simulink model "large_scale_autosar_swc_expfcns"  (R2021a)
settings: Solver=FixedStepDiscrete  StartTime=0.0  StopTime=20  FixedStep=1  MaxStep=.0001  RelTol=1e-3  EnableMultiTasking=on
undefined symbols (not defined in the file): DiscIntNeverNeededParam
(part 2 of 3)

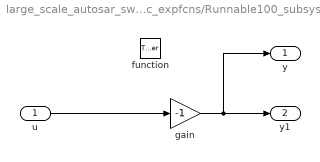
== system large_scale_autosar_swc_expfcns/Runnable100_subsystem ==
  u : Inport
  function : TriggerPort  TriggerType=function-call  VariantControl=Variant  SampleTimeType=periodic  SampleTime=-1
  gain : Gain  Gain=-1  ParamDataTypeStr=int8  OutDataTypeStr=int8
  y : Outport  InitialOutput=0  VectorParamsAs1DForOutWhenUnconnected=off
  y1 : Outport  Port=2  VectorParamsAs1DForOutWhenUnconnected=off
  wires:
  u/1 -> gain/1
  gain/1 -> y/1, y1/1

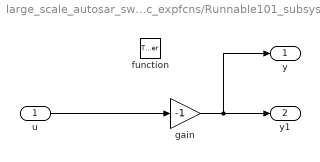
== system large_scale_autosar_swc_expfcns/Runnable101_subsystem ==
  u : Inport
  function : TriggerPort  TriggerType=function-call  VariantControl=Variant  SampleTimeType=periodic  SampleTime=-1
  gain : Gain  Gain=-1  ParamDataTypeStr=int8  OutDataTypeStr=int8
  y : Outport  InitialOutput=0  VectorParamsAs1DForOutWhenUnconnected=off
  y1 : Outport  Port=2  VectorParamsAs1DForOutWhenUnconnected=off
  wires:
  u/1 -> gain/1
  gain/1 -> y/1, y1/1

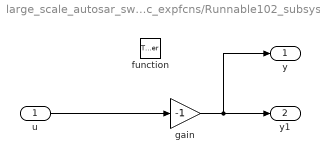
== system large_scale_autosar_swc_expfcns/Runnable102_subsystem ==
  u : Inport
  function : TriggerPort  TriggerType=function-call  VariantControl=Variant  SampleTimeType=periodic  SampleTime=-1
  gain : Gain  Gain=-1  ParamDataTypeStr=int8  OutDataTypeStr=int8
  y : Outport  InitialOutput=0  VectorParamsAs1DForOutWhenUnconnected=off
  y1 : Outport  Port=2  VectorParamsAs1DForOutWhenUnconnected=off
  wires:
  u/1 -> gain/1
  gain/1 -> y/1, y1/1

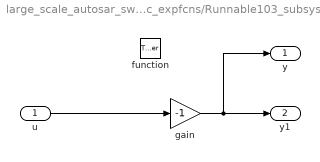
== system large_scale_autosar_swc_expfcns/Runnable103_subsystem ==
  u : Inport
  function : TriggerPort  TriggerType=function-call  VariantControl=Variant  SampleTimeType=periodic  SampleTime=-1
  gain : Gain  Gain=-1  ParamDataTypeStr=int8  OutDataTypeStr=int8
  y : Outport  InitialOutput=0  VectorParamsAs1DForOutWhenUnconnected=off
  y1 : Outport  Port=2  VectorParamsAs1DForOutWhenUnconnected=off
  wires:
  u/1 -> gain/1
  gain/1 -> y/1, y1/1

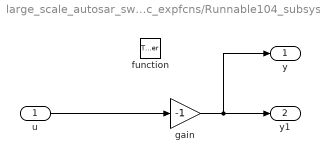
== system large_scale_autosar_swc_expfcns/Runnable104_subsystem ==
  u : Inport
  function : TriggerPort  TriggerType=function-call  VariantControl=Variant  SampleTimeType=periodic  SampleTime=-1
  gain : Gain  Gain=-1  ParamDataTypeStr=int8  OutDataTypeStr=int8
  y : Outport  InitialOutput=0  VectorParamsAs1DForOutWhenUnconnected=off
  y1 : Outport  Port=2  VectorParamsAs1DForOutWhenUnconnected=off
  wires:
  u/1 -> gain/1
  gain/1 -> y/1, y1/1

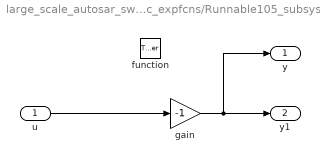
== system large_scale_autosar_swc_expfcns/Runnable105_subsystem ==
  u : Inport
  function : TriggerPort  TriggerType=function-call  VariantControl=Variant  SampleTimeType=periodic  SampleTime=-1
  gain : Gain  Gain=-1  ParamDataTypeStr=int8  OutDataTypeStr=int8
  y : Outport  InitialOutput=0  VectorParamsAs1DForOutWhenUnconnected=off
  y1 : Outport  Port=2  VectorParamsAs1DForOutWhenUnconnected=off
  wires:
  u/1 -> gain/1
  gain/1 -> y/1, y1/1

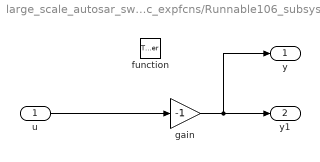
== system large_scale_autosar_swc_expfcns/Runnable106_subsystem ==
  u : Inport
  function : TriggerPort  TriggerType=function-call  VariantControl=Variant  SampleTimeType=periodic  SampleTime=-1
  gain : Gain  Gain=-1  ParamDataTypeStr=int8  OutDataTypeStr=int8
  y : Outport  InitialOutput=0  VectorParamsAs1DForOutWhenUnconnected=off
  y1 : Outport  Port=2  VectorParamsAs1DForOutWhenUnconnected=off
  wires:
  u/1 -> gain/1
  gain/1 -> y/1, y1/1

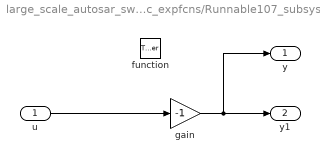
== system large_scale_autosar_swc_expfcns/Runnable107_subsystem ==
  u : Inport
  function : TriggerPort  TriggerType=function-call  VariantControl=Variant  SampleTimeType=periodic  SampleTime=-1
  gain : Gain  Gain=-1  ParamDataTypeStr=int8  OutDataTypeStr=int8
  y : Outport  InitialOutput=0  VectorParamsAs1DForOutWhenUnconnected=off
  y1 : Outport  Port=2  VectorParamsAs1DForOutWhenUnconnected=off
  wires:
  u/1 -> gain/1
  gain/1 -> y/1, y1/1

== system large_scale_autosar_swc_expfcns/Runnable108_subsystem ==
  u : Inport
  function : TriggerPort  TriggerType=function-call  VariantControl=Variant  SampleTimeType=periodic  SampleTime=-1
  gain : Gain  Gain=-1  ParamDataTypeStr=int8  OutDataTypeStr=int8
  y : Outport  InitialOutput=0  VectorParamsAs1DForOutWhenUnconnected=off
  y1 : Outport  Port=2  VectorParamsAs1DForOutWhenUnconnected=off
  wires:
  u/1 -> gain/1
  gain/1 -> y/1, y1/1

== system large_scale_autosar_swc_expfcns/Runnable10_subsystem ==
  u : Inport
  function : TriggerPort  TriggerType=function-call  VariantControl=Variant  SampleTimeType=periodic  SampleTime=-1
  gain : Gain  Gain=-1  ParamDataTypeStr=int8  OutDataTypeStr=int8
  y : Outport  InitialOutput=0  VectorParamsAs1DForOutWhenUnconnected=off
  y1 : Outport  Port=2  VectorParamsAs1DForOutWhenUnconnected=off
  wires:
  u/1 -> gain/1
  gain/1 -> y/1, y1/1

== system large_scale_autosar_swc_expfcns/Runnable11_subsystem ==
  u : Inport
  function : TriggerPort  TriggerType=function-call  VariantControl=Variant  SampleTimeType=periodic  SampleTime=-1
  gain : Gain  Gain=-1  ParamDataTypeStr=int8  OutDataTypeStr=int8
  y : Outport  InitialOutput=0  VectorParamsAs1DForOutWhenUnconnected=off
  y1 : Outport  Port=2  VectorParamsAs1DForOutWhenUnconnected=off
  wires:
  u/1 -> gain/1
  gain/1 -> y/1, y1/1

== system large_scale_autosar_swc_expfcns/Runnable12_subsystem ==
  u : Inport
  function : TriggerPort  TriggerType=function-call  VariantControl=Variant  SampleTimeType=periodic  SampleTime=-1
  gain : Gain  Gain=-1  ParamDataTypeStr=int8  OutDataTypeStr=int8
  y : Outport  InitialOutput=0  VectorParamsAs1DForOutWhenUnconnected=off
  y1 : Outport  Port=2  VectorParamsAs1DForOutWhenUnconnected=off
  wires:
  u/1 -> gain/1
  gain/1 -> y/1, y1/1

== system large_scale_autosar_swc_expfcns/Runnable13_subsystem ==
  u : Inport
  function : TriggerPort  TriggerType=function-call  VariantControl=Variant  SampleTimeType=periodic  SampleTime=-1
  gain : Gain  Gain=-1  ParamDataTypeStr=int8  OutDataTypeStr=int8
  y : Outport  InitialOutput=0  VectorParamsAs1DForOutWhenUnconnected=off
  y1 : Outport  Port=2  VectorParamsAs1DForOutWhenUnconnected=off
  wires:
  u/1 -> gain/1
  gain/1 -> y/1, y1/1

== system large_scale_autosar_swc_expfcns/Runnable14_subsystem ==
  u : Inport
  function : TriggerPort  TriggerType=function-call  VariantControl=Variant  SampleTimeType=periodic  SampleTime=-1
  gain : Gain  Gain=-1  ParamDataTypeStr=int8  OutDataTypeStr=int8
  y : Outport  InitialOutput=0  VectorParamsAs1DForOutWhenUnconnected=off
  y1 : Outport  Port=2  VectorParamsAs1DForOutWhenUnconnected=off
  wires:
  u/1 -> gain/1
  gain/1 -> y/1, y1/1

== system large_scale_autosar_swc_expfcns/Runnable15_subsystem ==
  u : Inport
  function : TriggerPort  TriggerType=function-call  VariantControl=Variant  SampleTimeType=periodic  SampleTime=-1
  gain : Gain  Gain=-1  ParamDataTypeStr=int8  OutDataTypeStr=int8
  y : Outport  InitialOutput=0  VectorParamsAs1DForOutWhenUnconnected=off
  y1 : Outport  Port=2  VectorParamsAs1DForOutWhenUnconnected=off
  wires:
  u/1 -> gain/1
  gain/1 -> y/1, y1/1

== system large_scale_autosar_swc_expfcns/Runnable16_subsystem ==
  u : Inport
  function : TriggerPort  TriggerType=function-call  VariantControl=Variant  SampleTimeType=periodic  SampleTime=-1
  gain : Gain  Gain=-1  ParamDataTypeStr=int8  OutDataTypeStr=int8
  y : Outport  InitialOutput=0  VectorParamsAs1DForOutWhenUnconnected=off
  y1 : Outport  Port=2  VectorParamsAs1DForOutWhenUnconnected=off
  wires:
  u/1 -> gain/1
  gain/1 -> y/1, y1/1

== system large_scale_autosar_swc_expfcns/Runnable17_subsystem ==
  u : Inport
  function : TriggerPort  TriggerType=function-call  VariantControl=Variant  SampleTimeType=periodic  SampleTime=-1
  gain : Gain  Gain=-1  ParamDataTypeStr=int8  OutDataTypeStr=int8
  y : Outport  InitialOutput=0  VectorParamsAs1DForOutWhenUnconnected=off
  y1 : Outport  Port=2  VectorParamsAs1DForOutWhenUnconnected=off
  wires:
  u/1 -> gain/1
  gain/1 -> y/1, y1/1

== system large_scale_autosar_swc_expfcns/Runnable18_subsystem ==
  u : Inport
  function : TriggerPort  TriggerType=function-call  VariantControl=Variant  SampleTimeType=periodic  SampleTime=-1
  gain : Gain  Gain=-1  ParamDataTypeStr=int8  OutDataTypeStr=int8
  y : Outport  InitialOutput=0  VectorParamsAs1DForOutWhenUnconnected=off
  y1 : Outport  Port=2  VectorParamsAs1DForOutWhenUnconnected=off
  wires:
  u/1 -> gain/1
  gain/1 -> y/1, y1/1

== system large_scale_autosar_swc_expfcns/Runnable19_subsystem ==
  u : Inport
  function : TriggerPort  TriggerType=function-call  VariantControl=Variant  SampleTimeType=periodic  SampleTime=-1
  gain : Gain  Gain=-1  ParamDataTypeStr=int8  OutDataTypeStr=int8
  y : Outport  InitialOutput=0  VectorParamsAs1DForOutWhenUnconnected=off
  y1 : Outport  Port=2  VectorParamsAs1DForOutWhenUnconnected=off
  wires:
  u/1 -> gain/1
  gain/1 -> y/1, y1/1

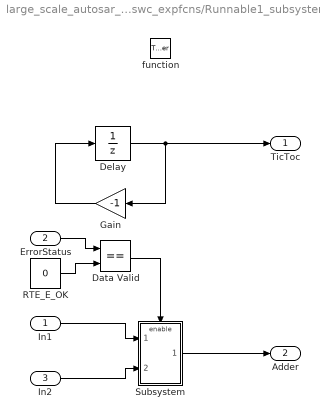
== system large_scale_autosar_swc_expfcns/Runnable1_subsystem ==
  In1 : Inport
  ErrorStatus : Inport  Port=2
  In2 : Inport  Port=3
  function : TriggerPort  TriggerType=function-call  VariantControl=Variant  SampleTimeType=periodic  SampleTime=-1
  Data Valid : RelationalOperator  Operator===  OutDataTypeStr=boolean  RndMeth=Nearest
  Delay : UnitDelay  InitialCondition=1  SampleTime=-1  HasFrameUpgradeWarning=on
  Gain : Gain  Gain=-1  OutDataTypeStr=fixdt(1,8,0)
  RTE_E_OK : Constant  Value=0
  Subsystem : Subsystem
  TicToc : Outport  InitialOutput=0  VectorParamsAs1DForOutWhenUnconnected=off
  Adder : Outport  Port=2  InitialOutput=0  VectorParamsAs1DForOutWhenUnconnected=off
  wires:
  RTE_E_OK/1 -> Data Valid/2
  ErrorStatus/1 -> Data Valid/1
  Data Valid/1 -> Subsystem/Enable
  In2/1 -> Subsystem/2(In2)
  In1/1 -> Subsystem/1(In1)
  Delay/1 -> Gain/1, TicToc/1
  Gain/1 -> Delay/1
  Subsystem/1(Adder) -> Adder/1

== system large_scale_autosar_swc_expfcns/Runnable20_subsystem ==
  u : Inport
  function : TriggerPort  TriggerType=function-call  VariantControl=Variant  SampleTimeType=periodic  SampleTime=-1
  gain : Gain  Gain=-1  ParamDataTypeStr=int8  OutDataTypeStr=int8
  y : Outport  InitialOutput=0  VectorParamsAs1DForOutWhenUnconnected=off
  y1 : Outport  Port=2  VectorParamsAs1DForOutWhenUnconnected=off
  wires:
  u/1 -> gain/1
  gain/1 -> y/1, y1/1

== system large_scale_autosar_swc_expfcns/Runnable21_subsystem ==
  u : Inport
  function : TriggerPort  TriggerType=function-call  VariantControl=Variant  SampleTimeType=periodic  SampleTime=-1
  gain : Gain  Gain=-1  ParamDataTypeStr=int8  OutDataTypeStr=int8
  y : Outport  InitialOutput=0  VectorParamsAs1DForOutWhenUnconnected=off
  y1 : Outport  Port=2  VectorParamsAs1DForOutWhenUnconnected=off
  wires:
  u/1 -> gain/1
  gain/1 -> y/1, y1/1

== system large_scale_autosar_swc_expfcns/Runnable22_subsystem ==
  u : Inport
  function : TriggerPort  TriggerType=function-call  VariantControl=Variant  SampleTimeType=periodic  SampleTime=-1
  gain : Gain  Gain=-1  ParamDataTypeStr=int8  OutDataTypeStr=int8
  y : Outport  InitialOutput=0  VectorParamsAs1DForOutWhenUnconnected=off
  y1 : Outport  Port=2  VectorParamsAs1DForOutWhenUnconnected=off
  wires:
  u/1 -> gain/1
  gain/1 -> y/1, y1/1

== system large_scale_autosar_swc_expfcns/Runnable23_subsystem ==
  u : Inport
  function : TriggerPort  TriggerType=function-call  VariantControl=Variant  SampleTimeType=periodic  SampleTime=-1
  gain : Gain  Gain=-1  ParamDataTypeStr=int8  OutDataTypeStr=int8
  y : Outport  InitialOutput=0  VectorParamsAs1DForOutWhenUnconnected=off
  y1 : Outport  Port=2  VectorParamsAs1DForOutWhenUnconnected=off
  wires:
  u/1 -> gain/1
  gain/1 -> y/1, y1/1

== system large_scale_autosar_swc_expfcns/Runnable24_subsystem ==
  u : Inport
  function : TriggerPort  TriggerType=function-call  VariantControl=Variant  SampleTimeType=periodic  SampleTime=-1
  gain : Gain  Gain=-1  ParamDataTypeStr=int8  OutDataTypeStr=int8
  y : Outport  InitialOutput=0  VectorParamsAs1DForOutWhenUnconnected=off
  y1 : Outport  Port=2  VectorParamsAs1DForOutWhenUnconnected=off
  wires:
  u/1 -> gain/1
  gain/1 -> y/1, y1/1

== system large_scale_autosar_swc_expfcns/Runnable25_subsystem ==
  u : Inport
  function : TriggerPort  TriggerType=function-call  VariantControl=Variant  SampleTimeType=periodic  SampleTime=-1
  gain : Gain  Gain=-1  ParamDataTypeStr=int8  OutDataTypeStr=int8
  y : Outport  InitialOutput=0  VectorParamsAs1DForOutWhenUnconnected=off
  y1 : Outport  Port=2  VectorParamsAs1DForOutWhenUnconnected=off
  wires:
  u/1 -> gain/1
  gain/1 -> y/1, y1/1

== system large_scale_autosar_swc_expfcns/Runnable26_subsystem ==
  u : Inport
  function : TriggerPort  TriggerType=function-call  VariantControl=Variant  SampleTimeType=periodic  SampleTime=-1
  gain : Gain  Gain=-1  ParamDataTypeStr=int8  OutDataTypeStr=int8
  y : Outport  InitialOutput=0  VectorParamsAs1DForOutWhenUnconnected=off
  y1 : Outport  Port=2  VectorParamsAs1DForOutWhenUnconnected=off
  wires:
  u/1 -> gain/1
  gain/1 -> y/1, y1/1

== system large_scale_autosar_swc_expfcns/Runnable27_subsystem ==
  u : Inport
  function : TriggerPort  TriggerType=function-call  VariantControl=Variant  SampleTimeType=periodic  SampleTime=-1
  gain : Gain  Gain=-1  ParamDataTypeStr=int8  OutDataTypeStr=int8
  y : Outport  InitialOutput=0  VectorParamsAs1DForOutWhenUnconnected=off
  y1 : Outport  Port=2  VectorParamsAs1DForOutWhenUnconnected=off
  wires:
  u/1 -> gain/1
  gain/1 -> y/1, y1/1

== system large_scale_autosar_swc_expfcns/Runnable28_subsystem ==
  u : Inport
  function : TriggerPort  TriggerType=function-call  VariantControl=Variant  SampleTimeType=periodic  SampleTime=-1
  gain : Gain  Gain=-1  ParamDataTypeStr=int8  OutDataTypeStr=int8
  y : Outport  InitialOutput=0  VectorParamsAs1DForOutWhenUnconnected=off
  y1 : Outport  Port=2  VectorParamsAs1DForOutWhenUnconnected=off
  wires:
  u/1 -> gain/1
  gain/1 -> y/1, y1/1

== system large_scale_autosar_swc_expfcns/Runnable29_subsystem ==
  u : Inport
  function : TriggerPort  TriggerType=function-call  VariantControl=Variant  SampleTimeType=periodic  SampleTime=-1
  gain : Gain  Gain=-1  ParamDataTypeStr=int8  OutDataTypeStr=int8
  y : Outport  InitialOutput=0  VectorParamsAs1DForOutWhenUnconnected=off
  y1 : Outport  Port=2  VectorParamsAs1DForOutWhenUnconnected=off
  wires:
  u/1 -> gain/1
  gain/1 -> y/1, y1/1

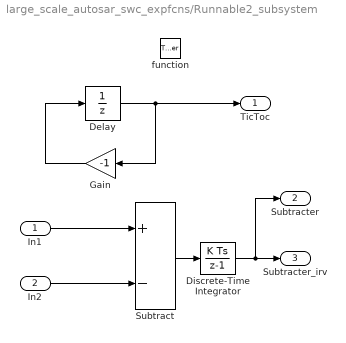
== system large_scale_autosar_swc_expfcns/Runnable2_subsystem ==
  In1 : Inport
  In2 : Inport  Port=2
  function : TriggerPort  TriggerType=function-call  VariantControl=Variant  SampleTimeType=periodic  SampleTime=-1
  Delay : UnitDelay  InitialCondition=1  SampleTime=-1  HasFrameUpgradeWarning=on
  Discrete-Time Integrator : DiscreteIntegrator  SampleTime=-1  ICPrevOutput=DiscIntNeverNeededParam  ICPrevScaledInput=DiscIntNeverNeededParam
  Gain : Gain  Gain=-1  OutDataTypeStr=fixdt(1,8,0)
  Subtract : Sum  Inputs=+-
  TicToc : Outport  InitialOutput=0  VectorParamsAs1DForOutWhenUnconnected=off
  Subtracter : Outport  Port=2  InitialOutput=0  VectorParamsAs1DForOutWhenUnconnected=off
  Subtracter_irv : Outport  Port=3  VectorParamsAs1DForOutWhenUnconnected=off
  wires:
  Discrete-Time Integrator/1 -> Subtracter/1, Subtracter_irv/1
  Subtract/1 -> Discrete-Time Integrator/1
  Gain/1 -> Delay/1
  Delay/1 -> TicToc/1, Gain/1
  In1/1 -> Subtract/1
  In2/1 -> Subtract/2

== system large_scale_autosar_swc_expfcns/Runnable30_subsystem ==
  u : Inport
  function : TriggerPort  TriggerType=function-call  VariantControl=Variant  SampleTimeType=periodic  SampleTime=-1
  gain : Gain  Gain=-1  ParamDataTypeStr=int8  OutDataTypeStr=int8
  y : Outport  InitialOutput=0  VectorParamsAs1DForOutWhenUnconnected=off
  y1 : Outport  Port=2  VectorParamsAs1DForOutWhenUnconnected=off
  wires:
  u/1 -> gain/1
  gain/1 -> y/1, y1/1

== system large_scale_autosar_swc_expfcns/Runnable31_subsystem ==
  u : Inport
  function : TriggerPort  TriggerType=function-call  VariantControl=Variant  SampleTimeType=periodic  SampleTime=-1
  gain : Gain  Gain=-1  ParamDataTypeStr=int8  OutDataTypeStr=int8
  y : Outport  InitialOutput=0  VectorParamsAs1DForOutWhenUnconnected=off
  y1 : Outport  Port=2  VectorParamsAs1DForOutWhenUnconnected=off
  wires:
  u/1 -> gain/1
  gain/1 -> y/1, y1/1

== system large_scale_autosar_swc_expfcns/Runnable32_subsystem ==
  u : Inport
  function : TriggerPort  TriggerType=function-call  VariantControl=Variant  SampleTimeType=periodic  SampleTime=-1
  gain : Gain  Gain=-1  ParamDataTypeStr=int8  OutDataTypeStr=int8
  y : Outport  InitialOutput=0  VectorParamsAs1DForOutWhenUnconnected=off
  y1 : Outport  Port=2  VectorParamsAs1DForOutWhenUnconnected=off
  wires:
  u/1 -> gain/1
  gain/1 -> y/1, y1/1

== system large_scale_autosar_swc_expfcns/Runnable33_subsystem ==
  u : Inport
  function : TriggerPort  TriggerType=function-call  VariantControl=Variant  SampleTimeType=periodic  SampleTime=-1
  gain : Gain  Gain=-1  ParamDataTypeStr=int8  OutDataTypeStr=int8
  y : Outport  InitialOutput=0  VectorParamsAs1DForOutWhenUnconnected=off
  y1 : Outport  Port=2  VectorParamsAs1DForOutWhenUnconnected=off
  wires:
  u/1 -> gain/1
  gain/1 -> y/1, y1/1

== system large_scale_autosar_swc_expfcns/Runnable34_subsystem ==
  u : Inport
  function : TriggerPort  TriggerType=function-call  VariantControl=Variant  SampleTimeType=periodic  SampleTime=-1
  gain : Gain  Gain=-1  ParamDataTypeStr=int8  OutDataTypeStr=int8
  y : Outport  InitialOutput=0  VectorParamsAs1DForOutWhenUnconnected=off
  y1 : Outport  Port=2  VectorParamsAs1DForOutWhenUnconnected=off
  wires:
  u/1 -> gain/1
  gain/1 -> y/1, y1/1

== system large_scale_autosar_swc_expfcns/Runnable35_subsystem ==
  u : Inport
  function : TriggerPort  TriggerType=function-call  VariantControl=Variant  SampleTimeType=periodic  SampleTime=-1
  gain : Gain  Gain=-1  ParamDataTypeStr=int8  OutDataTypeStr=int8
  y : Outport  InitialOutput=0  VectorParamsAs1DForOutWhenUnconnected=off
  y1 : Outport  Port=2  VectorParamsAs1DForOutWhenUnconnected=off
  wires:
  u/1 -> gain/1
  gain/1 -> y/1, y1/1

== system large_scale_autosar_swc_expfcns/Runnable36_subsystem ==
  u : Inport
  function : TriggerPort  TriggerType=function-call  VariantControl=Variant  SampleTimeType=periodic  SampleTime=-1
  gain : Gain  Gain=-1  ParamDataTypeStr=int8  OutDataTypeStr=int8
  y : Outport  InitialOutput=0  VectorParamsAs1DForOutWhenUnconnected=off
  y1 : Outport  Port=2  VectorParamsAs1DForOutWhenUnconnected=off
  wires:
  u/1 -> gain/1
  gain/1 -> y/1, y1/1

== system large_scale_autosar_swc_expfcns/Runnable37_subsystem ==
  u : Inport
  function : TriggerPort  TriggerType=function-call  VariantControl=Variant  SampleTimeType=periodic  SampleTime=-1
  gain : Gain  Gain=-1  ParamDataTypeStr=int8  OutDataTypeStr=int8
  y : Outport  InitialOutput=0  VectorParamsAs1DForOutWhenUnconnected=off
  y1 : Outport  Port=2  VectorParamsAs1DForOutWhenUnconnected=off
  wires:
  u/1 -> gain/1
  gain/1 -> y/1, y1/1

== system large_scale_autosar_swc_expfcns/Runnable38_subsystem ==
  u : Inport
  function : TriggerPort  TriggerType=function-call  VariantControl=Variant  SampleTimeType=periodic  SampleTime=-1
  gain : Gain  Gain=-1  ParamDataTypeStr=int8  OutDataTypeStr=int8
  y : Outport  InitialOutput=0  VectorParamsAs1DForOutWhenUnconnected=off
  y1 : Outport  Port=2  VectorParamsAs1DForOutWhenUnconnected=off
  wires:
  u/1 -> gain/1
  gain/1 -> y/1, y1/1

== system large_scale_autosar_swc_expfcns/Runnable39_subsystem ==
  u : Inport
  function : TriggerPort  TriggerType=function-call  VariantControl=Variant  SampleTimeType=periodic  SampleTime=-1
  gain : Gain  Gain=-1  ParamDataTypeStr=int8  OutDataTypeStr=int8
  y : Outport  InitialOutput=0  VectorParamsAs1DForOutWhenUnconnected=off
  y1 : Outport  Port=2  VectorParamsAs1DForOutWhenUnconnected=off
  wires:
  u/1 -> gain/1
  gain/1 -> y/1, y1/1

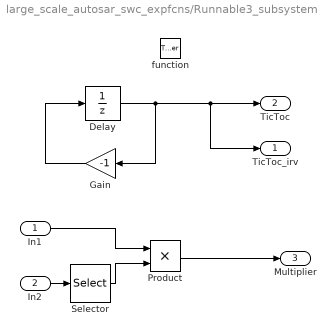
== system large_scale_autosar_swc_expfcns/Runnable3_subsystem ==
  In1 : Inport  OutDataTypeStr=double
  In2 : Inport  Port=2
  function : TriggerPort  TriggerType=function-call  VariantControl=Variant  SampleTimeType=periodic  SampleTime=-1
  Delay : UnitDelay  InitialCondition=1  SampleTime=-1  HasFrameUpgradeWarning=on
  Gain : Gain  Gain=-1  OutDataTypeStr=fixdt(1,8,0)
  Product : Product  Inputs=**  OutDataTypeStr=Inherit: Same as first input
  Selector : Selector  InputPortWidth=2  IndexOptions=Index vector (dialog)  Indices=1  OutputSizes=1
  TicToc_irv : Outport  VectorParamsAs1DForOutWhenUnconnected=off
  TicToc : Outport  Port=2  InitialOutput=0  VectorParamsAs1DForOutWhenUnconnected=off
  Multiplier : Outport  Port=3  InitialOutput=0  VectorParamsAs1DForOutWhenUnconnected=off
  wires:
  Selector/1 -> Product/2
  Product/1 -> Multiplier/1
  Gain/1 -> Delay/1
  Delay/1 -> TicToc_irv/1, TicToc/1, Gain/1
  In1/1 -> Product/1
  In2/1 -> Selector/1

== system large_scale_autosar_swc_expfcns/Runnable40_subsystem ==
  u : Inport
  function : TriggerPort  TriggerType=function-call  VariantControl=Variant  SampleTimeType=periodic  SampleTime=-1
  gain : Gain  Gain=-1  ParamDataTypeStr=int8  OutDataTypeStr=int8
  y : Outport  InitialOutput=0  VectorParamsAs1DForOutWhenUnconnected=off
  y1 : Outport  Port=2  VectorParamsAs1DForOutWhenUnconnected=off
  wires:
  u/1 -> gain/1
  gain/1 -> y/1, y1/1

== system large_scale_autosar_swc_expfcns/Runnable41_subsystem ==
  u : Inport
  function : TriggerPort  TriggerType=function-call  VariantControl=Variant  SampleTimeType=periodic  SampleTime=-1
  gain : Gain  Gain=-1  ParamDataTypeStr=int8  OutDataTypeStr=int8
  y : Outport  InitialOutput=0  VectorParamsAs1DForOutWhenUnconnected=off
  y1 : Outport  Port=2  VectorParamsAs1DForOutWhenUnconnected=off
  wires:
  u/1 -> gain/1
  gain/1 -> y/1, y1/1

== system large_scale_autosar_swc_expfcns/Runnable42_subsystem ==
  u : Inport
  function : TriggerPort  TriggerType=function-call  VariantControl=Variant  SampleTimeType=periodic  SampleTime=-1
  gain : Gain  Gain=-1  ParamDataTypeStr=int8  OutDataTypeStr=int8
  y : Outport  InitialOutput=0  VectorParamsAs1DForOutWhenUnconnected=off
  y1 : Outport  Port=2  VectorParamsAs1DForOutWhenUnconnected=off
  wires:
  u/1 -> gain/1
  gain/1 -> y/1, y1/1

== system large_scale_autosar_swc_expfcns/Runnable43_subsystem ==
  u : Inport
  function : TriggerPort  TriggerType=function-call  VariantControl=Variant  SampleTimeType=periodic  SampleTime=-1
  gain : Gain  Gain=-1  ParamDataTypeStr=int8  OutDataTypeStr=int8
  y : Outport  InitialOutput=0  VectorParamsAs1DForOutWhenUnconnected=off
  y1 : Outport  Port=2  VectorParamsAs1DForOutWhenUnconnected=off
  wires:
  u/1 -> gain/1
  gain/1 -> y/1, y1/1

== system large_scale_autosar_swc_expfcns/Runnable44_subsystem1 ==
  u : Inport
  function : TriggerPort  TriggerType=function-call  VariantControl=Variant  SampleTimeType=periodic  SampleTime=-1
  gain : Gain  Gain=-1  ParamDataTypeStr=int8  OutDataTypeStr=int8
  y : Outport  InitialOutput=0  VectorParamsAs1DForOutWhenUnconnected=off
  y1 : Outport  Port=2  VectorParamsAs1DForOutWhenUnconnected=off
  wires:
  u/1 -> gain/1
  gain/1 -> y/1, y1/1

== system large_scale_autosar_swc_expfcns/Runnable45_subsystem ==
  u : Inport
  function : TriggerPort  TriggerType=function-call  VariantControl=Variant  SampleTimeType=periodic  SampleTime=-1
  gain : Gain  Gain=-1  ParamDataTypeStr=int8  OutDataTypeStr=int8
  y : Outport  InitialOutput=0  VectorParamsAs1DForOutWhenUnconnected=off
  y1 : Outport  Port=2  VectorParamsAs1DForOutWhenUnconnected=off
  wires:
  u/1 -> gain/1
  gain/1 -> y/1, y1/1

== system large_scale_autosar_swc_expfcns/Runnable46_subsystem ==
  u : Inport
  function : TriggerPort  TriggerType=function-call  VariantControl=Variant  SampleTimeType=periodic  SampleTime=-1
  gain : Gain  Gain=-1  ParamDataTypeStr=int8  OutDataTypeStr=int8
  y : Outport  InitialOutput=0  VectorParamsAs1DForOutWhenUnconnected=off
  y1 : Outport  Port=2  VectorParamsAs1DForOutWhenUnconnected=off
  wires:
  u/1 -> gain/1
  gain/1 -> y/1, y1/1

== system large_scale_autosar_swc_expfcns/Runnable47_subsystem ==
  u : Inport
  function : TriggerPort  TriggerType=function-call  VariantControl=Variant  SampleTimeType=periodic  SampleTime=-1
  gain : Gain  Gain=-1  ParamDataTypeStr=int8  OutDataTypeStr=int8
  y : Outport  InitialOutput=0  VectorParamsAs1DForOutWhenUnconnected=off
  y1 : Outport  Port=2  VectorParamsAs1DForOutWhenUnconnected=off
  wires:
  u/1 -> gain/1
  gain/1 -> y/1, y1/1

== system large_scale_autosar_swc_expfcns/Runnable48_subsystem ==
  u : Inport
  function : TriggerPort  TriggerType=function-call  VariantControl=Variant  SampleTimeType=periodic  SampleTime=-1
  gain : Gain  Gain=-1  ParamDataTypeStr=int8  OutDataTypeStr=int8
  y : Outport  InitialOutput=0  VectorParamsAs1DForOutWhenUnconnected=off
  y1 : Outport  Port=2  VectorParamsAs1DForOutWhenUnconnected=off
  wires:
  u/1 -> gain/1
  gain/1 -> y/1, y1/1

== system large_scale_autosar_swc_expfcns/Runnable49_subsystem ==
  u : Inport
  function : TriggerPort  TriggerType=function-call  VariantControl=Variant  SampleTimeType=periodic  SampleTime=-1
  gain : Gain  Gain=-1  ParamDataTypeStr=int8  OutDataTypeStr=int8
  y : Outport  InitialOutput=0  VectorParamsAs1DForOutWhenUnconnected=off
  y1 : Outport  Port=2  VectorParamsAs1DForOutWhenUnconnected=off
  wires:
  u/1 -> gain/1
  gain/1 -> y/1, y1/1

== system large_scale_autosar_swc_expfcns/Runnable4_subsystem ==
  u : Inport
  function : TriggerPort  TriggerType=function-call  VariantControl=Variant  SampleTimeType=periodic  SampleTime=-1
  gain : Gain  Gain=-1  ParamDataTypeStr=int8  OutDataTypeStr=int8
  y : Outport  InitialOutput=0  VectorParamsAs1DForOutWhenUnconnected=off
  y1 : Outport  Port=2  VectorParamsAs1DForOutWhenUnconnected=off
  wires:
  u/1 -> gain/1
  gain/1 -> y/1, y1/1

== system large_scale_autosar_swc_expfcns/Runnable50_subsystem1 ==
  u : Inport
  function : TriggerPort  TriggerType=function-call  VariantControl=Variant  SampleTimeType=periodic  SampleTime=-1
  gain : Gain  Gain=-1  ParamDataTypeStr=int8  OutDataTypeStr=int8
  y : Outport  InitialOutput=0  VectorParamsAs1DForOutWhenUnconnected=off
  y1 : Outport  Port=2  VectorParamsAs1DForOutWhenUnconnected=off
  wires:
  u/1 -> gain/1
  gain/1 -> y/1, y1/1

== system large_scale_autosar_swc_expfcns/Runnable51_subsystem2 ==
  u : Inport
  function : TriggerPort  TriggerType=function-call  VariantControl=Variant  SampleTimeType=periodic  SampleTime=-1
  gain : Gain  Gain=-1  ParamDataTypeStr=int8  OutDataTypeStr=int8
  y : Outport  InitialOutput=0  VectorParamsAs1DForOutWhenUnconnected=off
  y1 : Outport  Port=2  VectorParamsAs1DForOutWhenUnconnected=off
  wires:
  u/1 -> gain/1
  gain/1 -> y/1, y1/1

== system large_scale_autosar_swc_expfcns/Runnable52_subsystem2 ==
  u : Inport
  function : TriggerPort  TriggerType=function-call  VariantControl=Variant  SampleTimeType=periodic  SampleTime=-1
  gain : Gain  Gain=-1  ParamDataTypeStr=int8  OutDataTypeStr=int8
  y : Outport  InitialOutput=0  VectorParamsAs1DForOutWhenUnconnected=off
  y1 : Outport  Port=2  VectorParamsAs1DForOutWhenUnconnected=off
  wires:
  u/1 -> gain/1
  gain/1 -> y/1, y1/1

== system large_scale_autosar_swc_expfcns/Runnable53_subsystem2 ==
  u : Inport
  function : TriggerPort  TriggerType=function-call  VariantControl=Variant  SampleTimeType=periodic  SampleTime=-1
  gain : Gain  Gain=-1  ParamDataTypeStr=int8  OutDataTypeStr=int8
  y : Outport  InitialOutput=0  VectorParamsAs1DForOutWhenUnconnected=off
  y1 : Outport  Port=2  VectorParamsAs1DForOutWhenUnconnected=off
  wires:
  u/1 -> gain/1
  gain/1 -> y/1, y1/1

== system large_scale_autosar_swc_expfcns/Runnable54_subsystem2 ==
  u : Inport
  function : TriggerPort  TriggerType=function-call  VariantControl=Variant  SampleTimeType=periodic  SampleTime=-1
  gain : Gain  Gain=-1  ParamDataTypeStr=int8  OutDataTypeStr=int8
  y : Outport  InitialOutput=0  VectorParamsAs1DForOutWhenUnconnected=off
  y1 : Outport  Port=2  VectorParamsAs1DForOutWhenUnconnected=off
  wires:
  u/1 -> gain/1
  gain/1 -> y/1, y1/1

== system large_scale_autosar_swc_expfcns/Runnable55_subsystem2 ==
  u : Inport
  function : TriggerPort  TriggerType=function-call  VariantControl=Variant  SampleTimeType=periodic  SampleTime=-1
  gain : Gain  Gain=-1  ParamDataTypeStr=int8  OutDataTypeStr=int8
  y : Outport  InitialOutput=0  VectorParamsAs1DForOutWhenUnconnected=off
  y1 : Outport  Port=2  VectorParamsAs1DForOutWhenUnconnected=off
  wires:
  u/1 -> gain/1
  gain/1 -> y/1, y1/1

== system large_scale_autosar_swc_expfcns/Runnable56_subsystem2 ==
  u : Inport
  function : TriggerPort  TriggerType=function-call  VariantControl=Variant  SampleTimeType=periodic  SampleTime=-1
  gain : Gain  Gain=-1  ParamDataTypeStr=int8  OutDataTypeStr=int8
  y : Outport  InitialOutput=0  VectorParamsAs1DForOutWhenUnconnected=off
  y1 : Outport  Port=2  VectorParamsAs1DForOutWhenUnconnected=off
  wires:
  u/1 -> gain/1
  gain/1 -> y/1, y1/1

== system large_scale_autosar_swc_expfcns/Runnable57_subsystem2 ==
  u : Inport
  function : TriggerPort  TriggerType=function-call  VariantControl=Variant  SampleTimeType=periodic  SampleTime=-1
  gain : Gain  Gain=-1  ParamDataTypeStr=int8  OutDataTypeStr=int8
  y : Outport  InitialOutput=0  VectorParamsAs1DForOutWhenUnconnected=off
  y1 : Outport  Port=2  VectorParamsAs1DForOutWhenUnconnected=off
  wires:
  u/1 -> gain/1
  gain/1 -> y/1, y1/1

== system large_scale_autosar_swc_expfcns/Runnable58_subsystem2 ==
  u : Inport
  function : TriggerPort  TriggerType=function-call  VariantControl=Variant  SampleTimeType=periodic  SampleTime=-1
  gain : Gain  Gain=-1  ParamDataTypeStr=int8  OutDataTypeStr=int8
  y : Outport  InitialOutput=0  VectorParamsAs1DForOutWhenUnconnected=off
  y1 : Outport  Port=2  VectorParamsAs1DForOutWhenUnconnected=off
  wires:
  u/1 -> gain/1
  gain/1 -> y/1, y1/1

== system large_scale_autosar_swc_expfcns/Runnable59_subsystem2 ==
  u : Inport
  function : TriggerPort  TriggerType=function-call  VariantControl=Variant  SampleTimeType=periodic  SampleTime=-1
  gain : Gain  Gain=-1  ParamDataTypeStr=int8  OutDataTypeStr=int8
  y : Outport  InitialOutput=0  VectorParamsAs1DForOutWhenUnconnected=off
  y1 : Outport  Port=2  VectorParamsAs1DForOutWhenUnconnected=off
  wires:
  u/1 -> gain/1
  gain/1 -> y/1, y1/1

== system large_scale_autosar_swc_expfcns/Runnable5_subsystem ==
  u : Inport
  function : TriggerPort  TriggerType=function-call  VariantControl=Variant  SampleTimeType=periodic  SampleTime=-1
  gain : Gain  Gain=-1  ParamDataTypeStr=int8  OutDataTypeStr=int8
  y : Outport  InitialOutput=0  VectorParamsAs1DForOutWhenUnconnected=off
  y1 : Outport  Port=2  VectorParamsAs1DForOutWhenUnconnected=off
  wires:
  u/1 -> gain/1
  gain/1 -> y/1, y1/1

== system large_scale_autosar_swc_expfcns/Runnable60_subsystem2 ==
  u : Inport
  function : TriggerPort  TriggerType=function-call  VariantControl=Variant  SampleTimeType=periodic  SampleTime=-1
  gain : Gain  Gain=-1  ParamDataTypeStr=int8  OutDataTypeStr=int8
  y : Outport  InitialOutput=0  VectorParamsAs1DForOutWhenUnconnected=off
  y1 : Outport  Port=2  VectorParamsAs1DForOutWhenUnconnected=off
  wires:
  u/1 -> gain/1
  gain/1 -> y/1, y1/1

== system large_scale_autosar_swc_expfcns/Runnable61_subsystem ==
  u : Inport
  function : TriggerPort  TriggerType=function-call  VariantControl=Variant  SampleTimeType=periodic  SampleTime=-1
  gain : Gain  Gain=-1  ParamDataTypeStr=int8  OutDataTypeStr=int8
  y : Outport  InitialOutput=0  VectorParamsAs1DForOutWhenUnconnected=off
  y1 : Outport  Port=2  VectorParamsAs1DForOutWhenUnconnected=off
  wires:
  u/1 -> gain/1
  gain/1 -> y/1, y1/1

== system large_scale_autosar_swc_expfcns/Runnable62_subsystem ==
  u : Inport
  function : TriggerPort  TriggerType=function-call  VariantControl=Variant  SampleTimeType=periodic  SampleTime=-1
  gain : Gain  Gain=-1  ParamDataTypeStr=int8  OutDataTypeStr=int8
  y : Outport  InitialOutput=0  VectorParamsAs1DForOutWhenUnconnected=off
  y1 : Outport  Port=2  VectorParamsAs1DForOutWhenUnconnected=off
  wires:
  u/1 -> gain/1
  gain/1 -> y/1, y1/1

== system large_scale_autosar_swc_expfcns/Runnable63_subsystem ==
  u : Inport
  function : TriggerPort  TriggerType=function-call  VariantControl=Variant  SampleTimeType=periodic  SampleTime=-1
  gain : Gain  Gain=-1  ParamDataTypeStr=int8  OutDataTypeStr=int8
  y : Outport  InitialOutput=0  VectorParamsAs1DForOutWhenUnconnected=off
  y1 : Outport  Port=2  VectorParamsAs1DForOutWhenUnconnected=off
  wires:
  u/1 -> gain/1
  gain/1 -> y/1, y1/1

== system large_scale_autosar_swc_expfcns/Runnable64_subsystem ==
  u : Inport
  function : TriggerPort  TriggerType=function-call  VariantControl=Variant  SampleTimeType=periodic  SampleTime=-1
  gain : Gain  Gain=-1  ParamDataTypeStr=int8  OutDataTypeStr=int8
  y : Outport  InitialOutput=0  VectorParamsAs1DForOutWhenUnconnected=off
  y1 : Outport  Port=2  VectorParamsAs1DForOutWhenUnconnected=off
  wires:
  u/1 -> gain/1
  gain/1 -> y/1, y1/1

== system large_scale_autosar_swc_expfcns/Runnable65_subsystem ==
  u : Inport
  function : TriggerPort  TriggerType=function-call  VariantControl=Variant  SampleTimeType=periodic  SampleTime=-1
  gain : Gain  Gain=-1  ParamDataTypeStr=int8  OutDataTypeStr=int8
  y : Outport  InitialOutput=0  VectorParamsAs1DForOutWhenUnconnected=off
  y1 : Outport  Port=2  VectorParamsAs1DForOutWhenUnconnected=off
  wires:
  u/1 -> gain/1
  gain/1 -> y/1, y1/1

== system large_scale_autosar_swc_expfcns/Runnable66_subsystem3 ==
  u : Inport
  function : TriggerPort  TriggerType=function-call  VariantControl=Variant  SampleTimeType=periodic  SampleTime=-1
  gain : Gain  Gain=-1  ParamDataTypeStr=int8  OutDataTypeStr=int8
  y : Outport  InitialOutput=0  VectorParamsAs1DForOutWhenUnconnected=off
  y1 : Outport  Port=2  VectorParamsAs1DForOutWhenUnconnected=off
  wires:
  u/1 -> gain/1
  gain/1 -> y/1, y1/1

== system large_scale_autosar_swc_expfcns/Runnable67_subsystem ==
  u : Inport
  function : TriggerPort  TriggerType=function-call  VariantControl=Variant  SampleTimeType=periodic  SampleTime=-1
  gain : Gain  Gain=-1  ParamDataTypeStr=int8  OutDataTypeStr=int8
  y : Outport  InitialOutput=0  VectorParamsAs1DForOutWhenUnconnected=off
  y1 : Outport  Port=2  VectorParamsAs1DForOutWhenUnconnected=off
  wires:
  u/1 -> gain/1
  gain/1 -> y/1, y1/1

== system large_scale_autosar_swc_expfcns/Runnable68_subsystem ==
  u : Inport
  function : TriggerPort  TriggerType=function-call  VariantControl=Variant  SampleTimeType=periodic  SampleTime=-1
  gain : Gain  Gain=-1  ParamDataTypeStr=int8  OutDataTypeStr=int8
  y : Outport  InitialOutput=0  VectorParamsAs1DForOutWhenUnconnected=off
  y1 : Outport  Port=2  VectorParamsAs1DForOutWhenUnconnected=off
  wires:
  u/1 -> gain/1
  gain/1 -> y/1, y1/1

== system large_scale_autosar_swc_expfcns/Runnable69_subsystem ==
  u : Inport
  function : TriggerPort  TriggerType=function-call  VariantControl=Variant  SampleTimeType=periodic  SampleTime=-1
  gain : Gain  Gain=-1  ParamDataTypeStr=int8  OutDataTypeStr=int8
  y : Outport  InitialOutput=0  VectorParamsAs1DForOutWhenUnconnected=off
  y1 : Outport  Port=2  VectorParamsAs1DForOutWhenUnconnected=off
  wires:
  u/1 -> gain/1
  gain/1 -> y/1, y1/1

== system large_scale_autosar_swc_expfcns/Runnable6_subsystem ==
  u : Inport
  function : TriggerPort  TriggerType=function-call  VariantControl=Variant  SampleTimeType=periodic  SampleTime=-1
  gain : Gain  Gain=-1  ParamDataTypeStr=int8  OutDataTypeStr=int8
  y : Outport  InitialOutput=0  VectorParamsAs1DForOutWhenUnconnected=off
  y1 : Outport  Port=2  VectorParamsAs1DForOutWhenUnconnected=off
  wires:
  u/1 -> gain/1
  gain/1 -> y/1, y1/1

== system large_scale_autosar_swc_expfcns/Runnable70_subsystem ==
  u : Inport
  function : TriggerPort  TriggerType=function-call  VariantControl=Variant  SampleTimeType=periodic  SampleTime=-1
  gain : Gain  Gain=-1  ParamDataTypeStr=int8  OutDataTypeStr=int8
  y : Outport  InitialOutput=0  VectorParamsAs1DForOutWhenUnconnected=off
  y1 : Outport  Port=2  VectorParamsAs1DForOutWhenUnconnected=off
  wires:
  u/1 -> gain/1
  gain/1 -> y/1, y1/1

== system large_scale_autosar_swc_expfcns/Runnable71_subsystem ==
  u : Inport
  function : TriggerPort  TriggerType=function-call  VariantControl=Variant  SampleTimeType=periodic  SampleTime=-1
  gain : Gain  Gain=-1  ParamDataTypeStr=int8  OutDataTypeStr=int8
  y : Outport  InitialOutput=0  VectorParamsAs1DForOutWhenUnconnected=off
  y1 : Outport  Port=2  VectorParamsAs1DForOutWhenUnconnected=off
  wires:
  u/1 -> gain/1
  gain/1 -> y/1, y1/1

== system large_scale_autosar_swc_expfcns/Runnable72_subsystem ==
  u : Inport
  function : TriggerPort  TriggerType=function-call  VariantControl=Variant  SampleTimeType=periodic  SampleTime=-1
  gain : Gain  Gain=-1  ParamDataTypeStr=int8  OutDataTypeStr=int8
  y : Outport  InitialOutput=0  VectorParamsAs1DForOutWhenUnconnected=off
  y1 : Outport  Port=2  VectorParamsAs1DForOutWhenUnconnected=off
  wires:
  u/1 -> gain/1
  gain/1 -> y/1, y1/1

== system large_scale_autosar_swc_expfcns/Runnable73_subsystem ==
  u : Inport
  function : TriggerPort  TriggerType=function-call  VariantControl=Variant  SampleTimeType=periodic  SampleTime=-1
  gain : Gain  Gain=-1  ParamDataTypeStr=int8  OutDataTypeStr=int8
  y : Outport  InitialOutput=0  VectorParamsAs1DForOutWhenUnconnected=off
  y1 : Outport  Port=2  VectorParamsAs1DForOutWhenUnconnected=off
  wires:
  u/1 -> gain/1
  gain/1 -> y/1, y1/1

== system large_scale_autosar_swc_expfcns/Runnable74_subsystem ==
  u : Inport
  function : TriggerPort  TriggerType=function-call  VariantControl=Variant  SampleTimeType=periodic  SampleTime=-1
  gain : Gain  Gain=-1  ParamDataTypeStr=int8  OutDataTypeStr=int8
  y : Outport  InitialOutput=0  VectorParamsAs1DForOutWhenUnconnected=off
  y1 : Outport  Port=2  VectorParamsAs1DForOutWhenUnconnected=off
  wires:
  u/1 -> gain/1
  gain/1 -> y/1, y1/1

== system large_scale_autosar_swc_expfcns/Runnable75_subsystem ==
  u : Inport
  function : TriggerPort  TriggerType=function-call  VariantControl=Variant  SampleTimeType=periodic  SampleTime=-1
  gain : Gain  Gain=-1  ParamDataTypeStr=int8  OutDataTypeStr=int8
  y : Outport  InitialOutput=0  VectorParamsAs1DForOutWhenUnconnected=off
  y1 : Outport  Port=2  VectorParamsAs1DForOutWhenUnconnected=off
  wires:
  u/1 -> gain/1
  gain/1 -> y/1, y1/1

== system large_scale_autosar_swc_expfcns/Runnable76_subsystem ==
  u : Inport
  function : TriggerPort  TriggerType=function-call  VariantControl=Variant  SampleTimeType=periodic  SampleTime=-1
  gain : Gain  Gain=-1  ParamDataTypeStr=int8  OutDataTypeStr=int8
  y : Outport  InitialOutput=0  VectorParamsAs1DForOutWhenUnconnected=off
  y1 : Outport  Port=2  VectorParamsAs1DForOutWhenUnconnected=off
  wires:
  u/1 -> gain/1
  gain/1 -> y/1, y1/1

== system large_scale_autosar_swc_expfcns/Runnable77_subsystem ==
  u : Inport
  function : TriggerPort  TriggerType=function-call  VariantControl=Variant  SampleTimeType=periodic  SampleTime=-1
  gain : Gain  Gain=-1  ParamDataTypeStr=int8  OutDataTypeStr=int8
  y : Outport  InitialOutput=0  VectorParamsAs1DForOutWhenUnconnected=off
  y1 : Outport  Port=2  VectorParamsAs1DForOutWhenUnconnected=off
  wires:
  u/1 -> gain/1
  gain/1 -> y/1, y1/1

== system large_scale_autosar_swc_expfcns/Runnable78_subsystem ==
  u : Inport
  function : TriggerPort  TriggerType=function-call  VariantControl=Variant  SampleTimeType=periodic  SampleTime=-1
  gain : Gain  Gain=-1  ParamDataTypeStr=int8  OutDataTypeStr=int8
  y : Outport  InitialOutput=0  VectorParamsAs1DForOutWhenUnconnected=off
  y1 : Outport  Port=2  VectorParamsAs1DForOutWhenUnconnected=off
  wires:
  u/1 -> gain/1
  gain/1 -> y/1, y1/1

== system large_scale_autosar_swc_expfcns/Runnable79_subsystem ==
  u : Inport
  function : TriggerPort  TriggerType=function-call  VariantControl=Variant  SampleTimeType=periodic  SampleTime=-1
  gain : Gain  Gain=-1  ParamDataTypeStr=int8  OutDataTypeStr=int8
  y : Outport  InitialOutput=0  VectorParamsAs1DForOutWhenUnconnected=off
  y1 : Outport  Port=2  VectorParamsAs1DForOutWhenUnconnected=off
  wires:
  u/1 -> gain/1
  gain/1 -> y/1, y1/1

== system large_scale_autosar_swc_expfcns/Runnable7_subsystem ==
  u : Inport
  function : TriggerPort  TriggerType=function-call  VariantControl=Variant  SampleTimeType=periodic  SampleTime=-1
  gain : Gain  Gain=-1  ParamDataTypeStr=int8  OutDataTypeStr=int8
  y : Outport  InitialOutput=0  VectorParamsAs1DForOutWhenUnconnected=off
  y1 : Outport  Port=2  VectorParamsAs1DForOutWhenUnconnected=off
  wires:
  u/1 -> gain/1
  gain/1 -> y/1, y1/1

== system large_scale_autosar_swc_expfcns/Runnable80_subsystem ==
  u : Inport
  function : TriggerPort  TriggerType=function-call  VariantControl=Variant  SampleTimeType=periodic  SampleTime=-1
  gain : Gain  Gain=-1  ParamDataTypeStr=int8  OutDataTypeStr=int8
  y : Outport  InitialOutput=0  VectorParamsAs1DForOutWhenUnconnected=off
  y1 : Outport  Port=2  VectorParamsAs1DForOutWhenUnconnected=off
  wires:
  u/1 -> gain/1
  gain/1 -> y/1, y1/1

== system large_scale_autosar_swc_expfcns/Runnable81_subsystem ==
  u : Inport
  function : TriggerPort  TriggerType=function-call  VariantControl=Variant  SampleTimeType=periodic  SampleTime=-1
  gain : Gain  Gain=-1  ParamDataTypeStr=int8  OutDataTypeStr=int8
  y : Outport  InitialOutput=0  VectorParamsAs1DForOutWhenUnconnected=off
  y1 : Outport  Port=2  VectorParamsAs1DForOutWhenUnconnected=off
  wires:
  u/1 -> gain/1
  gain/1 -> y/1, y1/1

== system large_scale_autosar_swc_expfcns/Runnable82_subsystem ==
  u : Inport
  function : TriggerPort  TriggerType=function-call  VariantControl=Variant  SampleTimeType=periodic  SampleTime=-1
  gain : Gain  Gain=-1  ParamDataTypeStr=int8  OutDataTypeStr=int8
  y : Outport  InitialOutput=0  VectorParamsAs1DForOutWhenUnconnected=off
  y1 : Outport  Port=2  VectorParamsAs1DForOutWhenUnconnected=off
  wires:
  u/1 -> gain/1
  gain/1 -> y/1, y1/1

== system large_scale_autosar_swc_expfcns/Runnable83_subsystem ==
  u : Inport
  function : TriggerPort  TriggerType=function-call  VariantControl=Variant  SampleTimeType=periodic  SampleTime=-1
  gain : Gain  Gain=-1  ParamDataTypeStr=int8  OutDataTypeStr=int8
  y : Outport  InitialOutput=0  VectorParamsAs1DForOutWhenUnconnected=off
  y1 : Outport  Port=2  VectorParamsAs1DForOutWhenUnconnected=off
  wires:
  u/1 -> gain/1
  gain/1 -> y/1, y1/1

== system large_scale_autosar_swc_expfcns/Runnable84_subsystem ==
  u : Inport
  function : TriggerPort  TriggerType=function-call  VariantControl=Variant  SampleTimeType=periodic  SampleTime=-1
  gain : Gain  Gain=-1  ParamDataTypeStr=int8  OutDataTypeStr=int8
  y : Outport  InitialOutput=0  VectorParamsAs1DForOutWhenUnconnected=off
  y1 : Outport  Port=2  VectorParamsAs1DForOutWhenUnconnected=off
  wires:
  u/1 -> gain/1
  gain/1 -> y/1, y1/1

== system large_scale_autosar_swc_expfcns/Runnable85_subsystem ==
  u : Inport
  function : TriggerPort  TriggerType=function-call  VariantControl=Variant  SampleTimeType=periodic  SampleTime=-1
  gain : Gain  Gain=-1  ParamDataTypeStr=int8  OutDataTypeStr=int8
  y : Outport  InitialOutput=0  VectorParamsAs1DForOutWhenUnconnected=off
  y1 : Outport  Port=2  VectorParamsAs1DForOutWhenUnconnected=off
  wires:
  u/1 -> gain/1
  gain/1 -> y/1, y1/1

== system large_scale_autosar_swc_expfcns/Runnable86_subsystem ==
  u : Inport
  function : TriggerPort  TriggerType=function-call  VariantControl=Variant  SampleTimeType=periodic  SampleTime=-1
  gain : Gain  Gain=-1  ParamDataTypeStr=int8  OutDataTypeStr=int8
  y : Outport  InitialOutput=0  VectorParamsAs1DForOutWhenUnconnected=off
  y1 : Outport  Port=2  VectorParamsAs1DForOutWhenUnconnected=off
  wires:
  u/1 -> gain/1
  gain/1 -> y/1, y1/1

== system large_scale_autosar_swc_expfcns/Runnable87_subsystem ==
  u : Inport
  function : TriggerPort  TriggerType=function-call  VariantControl=Variant  SampleTimeType=periodic  SampleTime=-1
  gain : Gain  Gain=-1  ParamDataTypeStr=int8  OutDataTypeStr=int8
  y : Outport  InitialOutput=0  VectorParamsAs1DForOutWhenUnconnected=off
  y1 : Outport  Port=2  VectorParamsAs1DForOutWhenUnconnected=off
  wires:
  u/1 -> gain/1
  gain/1 -> y/1, y1/1

== system large_scale_autosar_swc_expfcns/Runnable88_subsystem ==
  u : Inport
  function : TriggerPort  TriggerType=function-call  VariantControl=Variant  SampleTimeType=periodic  SampleTime=-1
  gain : Gain  Gain=-1  ParamDataTypeStr=int8  OutDataTypeStr=int8
  y : Outport  InitialOutput=0  VectorParamsAs1DForOutWhenUnconnected=off
  y1 : Outport  Port=2  VectorParamsAs1DForOutWhenUnconnected=off
  wires:
  u/1 -> gain/1
  gain/1 -> y/1, y1/1

== system large_scale_autosar_swc_expfcns/Runnable89_subsystem ==
  u : Inport
  function : TriggerPort  TriggerType=function-call  VariantControl=Variant  SampleTimeType=periodic  SampleTime=-1
  gain : Gain  Gain=-1  ParamDataTypeStr=int8  OutDataTypeStr=int8
  y : Outport  InitialOutput=0  VectorParamsAs1DForOutWhenUnconnected=off
  y1 : Outport  Port=2  VectorParamsAs1DForOutWhenUnconnected=off
  wires:
  u/1 -> gain/1
  gain/1 -> y/1, y1/1

== system large_scale_autosar_swc_expfcns/Runnable8_subsystem ==
  u : Inport
  function : TriggerPort  TriggerType=function-call  VariantControl=Variant  SampleTimeType=periodic  SampleTime=-1
  gain : Gain  Gain=-1  ParamDataTypeStr=int8  OutDataTypeStr=int8
  y : Outport  InitialOutput=0  VectorParamsAs1DForOutWhenUnconnected=off
  y1 : Outport  Port=2  VectorParamsAs1DForOutWhenUnconnected=off
  wires:
  u/1 -> gain/1
  gain/1 -> y/1, y1/1

== system large_scale_autosar_swc_expfcns/Runnable90_subsystem ==
  u : Inport
  function : TriggerPort  TriggerType=function-call  VariantControl=Variant  SampleTimeType=periodic  SampleTime=-1
  gain : Gain  Gain=-1  ParamDataTypeStr=int8  OutDataTypeStr=int8
  y : Outport  InitialOutput=0  VectorParamsAs1DForOutWhenUnconnected=off
  y1 : Outport  Port=2  VectorParamsAs1DForOutWhenUnconnected=off
  wires:
  u/1 -> gain/1
  gain/1 -> y/1, y1/1

== system large_scale_autosar_swc_expfcns/Runnable91_subsystem ==
  u : Inport
  function : TriggerPort  TriggerType=function-call  VariantControl=Variant  SampleTimeType=periodic  SampleTime=-1
  gain : Gain  Gain=-1  ParamDataTypeStr=int8  OutDataTypeStr=int8
  y : Outport  InitialOutput=0  VectorParamsAs1DForOutWhenUnconnected=off
  y1 : Outport  Port=2  VectorParamsAs1DForOutWhenUnconnected=off
  wires:
  u/1 -> gain/1
  gain/1 -> y/1, y1/1

== system large_scale_autosar_swc_expfcns/Runnable92_subsystem6 ==
  u : Inport
  function : TriggerPort  TriggerType=function-call  VariantControl=Variant  SampleTimeType=periodic  SampleTime=-1
  gain : Gain  Gain=-1  ParamDataTypeStr=int8  OutDataTypeStr=int8
  y : Outport  InitialOutput=0  VectorParamsAs1DForOutWhenUnconnected=off
  y1 : Outport  Port=2  VectorParamsAs1DForOutWhenUnconnected=off
  wires:
  u/1 -> gain/1
  gain/1 -> y/1, y1/1

== system large_scale_autosar_swc_expfcns/Runnable93_subsystem ==
  u : Inport
  function : TriggerPort  TriggerType=function-call  VariantControl=Variant  SampleTimeType=periodic  SampleTime=-1
  gain : Gain  Gain=-1  ParamDataTypeStr=int8  OutDataTypeStr=int8
  y : Outport  InitialOutput=0  VectorParamsAs1DForOutWhenUnconnected=off
  y1 : Outport  Port=2  VectorParamsAs1DForOutWhenUnconnected=off
  wires:
  u/1 -> gain/1
  gain/1 -> y/1, y1/1

== system large_scale_autosar_swc_expfcns/Runnable94_subsystem ==
  u : Inport
  function : TriggerPort  TriggerType=function-call  VariantControl=Variant  SampleTimeType=periodic  SampleTime=-1
  gain : Gain  Gain=-1  ParamDataTypeStr=int8  OutDataTypeStr=int8
  y : Outport  InitialOutput=0  VectorParamsAs1DForOutWhenUnconnected=off
  y1 : Outport  Port=2  VectorParamsAs1DForOutWhenUnconnected=off
  wires:
  u/1 -> gain/1
  gain/1 -> y/1, y1/1

== system large_scale_autosar_swc_expfcns/Runnable95_subsystem ==
  u : Inport
  function : TriggerPort  TriggerType=function-call  VariantControl=Variant  SampleTimeType=periodic  SampleTime=-1
  gain : Gain  Gain=-1  ParamDataTypeStr=int8  OutDataTypeStr=int8
  y : Outport  InitialOutput=0  VectorParamsAs1DForOutWhenUnconnected=off
  y1 : Outport  Port=2  VectorParamsAs1DForOutWhenUnconnected=off
  wires:
  u/1 -> gain/1
  gain/1 -> y/1, y1/1

== system large_scale_autosar_swc_expfcns/Runnable96_subsystem ==
  u : Inport
  function : TriggerPort  TriggerType=function-call  VariantControl=Variant  SampleTimeType=periodic  SampleTime=-1
  gain : Gain  Gain=-1  ParamDataTypeStr=int8  OutDataTypeStr=int8
  y : Outport  InitialOutput=0  VectorParamsAs1DForOutWhenUnconnected=off
  y1 : Outport  Port=2  VectorParamsAs1DForOutWhenUnconnected=off
  wires:
  u/1 -> gain/1
  gain/1 -> y/1, y1/1

== system large_scale_autosar_swc_expfcns/Runnable97_subsystem ==
  u : Inport
  function : TriggerPort  TriggerType=function-call  VariantControl=Variant  SampleTimeType=periodic  SampleTime=-1
  gain : Gain  Gain=-1  ParamDataTypeStr=int8  OutDataTypeStr=int8
  y : Outport  InitialOutput=0  VectorParamsAs1DForOutWhenUnconnected=off
  y1 : Outport  Port=2  VectorParamsAs1DForOutWhenUnconnected=off
  wires:
  u/1 -> gain/1
  gain/1 -> y/1, y1/1
